simulink model "HQEV_MiL_20160830_integrate_r2017a_testframe"  (R2017a)
settings: Solver=FixedStepDiscrete  StartTime=0.0  StopTime=inf  FixedStep=0.01  RelTol=1e-3  EnableMultiTasking=on
PreLoadFcn:
  | try
  | load('HQEV_MiL_20160830_integrate_r2017a_testframe_tpt_so.mat');
  | catch
  | error('Could not load the file HQEV_MiL_20160830_integrate_r2017a_testframe_tpt_so.mat. This file contains Simulink objects that are possibly required for executing the test frame model. Try re-generating the test frame model.');
  | end
PostLoadFcn:
  | , if any(exist('dsrtsu_mdlpostloadfcn', 'file') == [2, 3, 6]), try dsrtsu_mdlpostloadfcn('Execute', bdroot); catch fprintf('Error in PostLoadFcn (dsrtsu_mdlpostloadfcn) for model "%s":\n %s\n', bdroot, lasterr); end, end,
values from neighbouring files (symbols this model uses):
  tpt_stepsize = builtin('double',0.01)    [HQEV_MiL_20160830_integrate_r20_tpt_io.m]
undefined symbols (not defined in the file or in its folder): pPUD_cnt_ACChItErrThd_C, pPUD_cnt_ACHeatItErrThd_C, pPUD_cnt_DCChItErrThd_C, pPUD_cnt_DCHeatItErrThd_C, pPUD_s_ACChrg1NoRespTiout_C, pPUD_s_ACChrg2NoRespTiout_C, pPUD_s_ACChrgPtcEnDly_C, pPUD_s_BMSOnNoRespTiout_C, pPUD_s_DCChrg1NoRespTiout_C, pPUD_s_DCChrg2NoRespTiout_C, pPUD_s_EgyCoorrChItRecoverDly_C, pPUD_s_EgyCoorrDlyRstCtr_C, pPUD_s_EgyCoorrNoRespTiout_C, pPUD_V_MotPwrVolt_C, pPUD_V_MotRpdDisVolt_C, PUD, PUD_lib
libraries: BaseOperationLib_Browser x22, simulink x1, tpt_sfun_lib x1
settings Model: Creator=wuaibin  LastModifiedBy=YangFuchun
settings DataIOCC: LimitDataPoints=on  SaveFormat=StructureWithTime  SignalLoggingSaveFormat=ModelDataLogs
settings OptimizationCC: BlockReduction=off  UseFloatMulNetSlope=on  DefaultUnderspecifiedDataType=single  ExpressionDepthLimit=2147483647  LifeSpan=inf
settings DebuggingCC: UnderspecifiedInitializationDetection=Classic  MergeDetectMultiDrivingBlocksExec=none  SolverPrmCheckMsg=warning  FcnCallInpInsideContextMsg=warning  StateNameClashWarn=warning  StrictBusMsg=ErrorOnBusTreatedAsVector  NonBusSignalsTreatedAsBus=error  SFUnexpectedBacktrackingDiag=warning  SFNoUnconditionalDefaultTransitionDiag=warning  SFExecutionAtInitializationDiag=none
settings HardwareCC: ProdBitPerPointer=32  ProdBitPerSizeT=32  ProdBitPerPtrDiffT=32  ProdLargestAtomicFloat=None  ProdEndianess=BigEndian  ProdWordSize=32  ProdHWDeviceType=Generic->Custom  TargetIntDivRoundTo=Zero  TargetEndianess=BigEndian  TargetHWDeviceType=Generic->Custom
settings ModelReferenceCC: PropagateSignalLabelsOutOfModel=off
settings RTWCC: GenerateMakefile=off  TemplateMakefile=grt_msvc.tmf  Description="Visual C/C++ Project Makefile only for the \"grt\" target"
settings GRTTargetCC: TargetLangStandard=C89/C90 (ANSI)  GeneratePreprocessorConditionals=Disable all  CombineOutputUpdateFcns=off  GRTInterface=on
settings ConfigComp: CovMetricSettings=dw  CovHtmlReporting=on  CovSaveCumulativeToWorkspaceVar=on  CovSaveSingleToWorkspaceVar=on  CovExternalEMLEnable=off  CovSFcnEnable=off

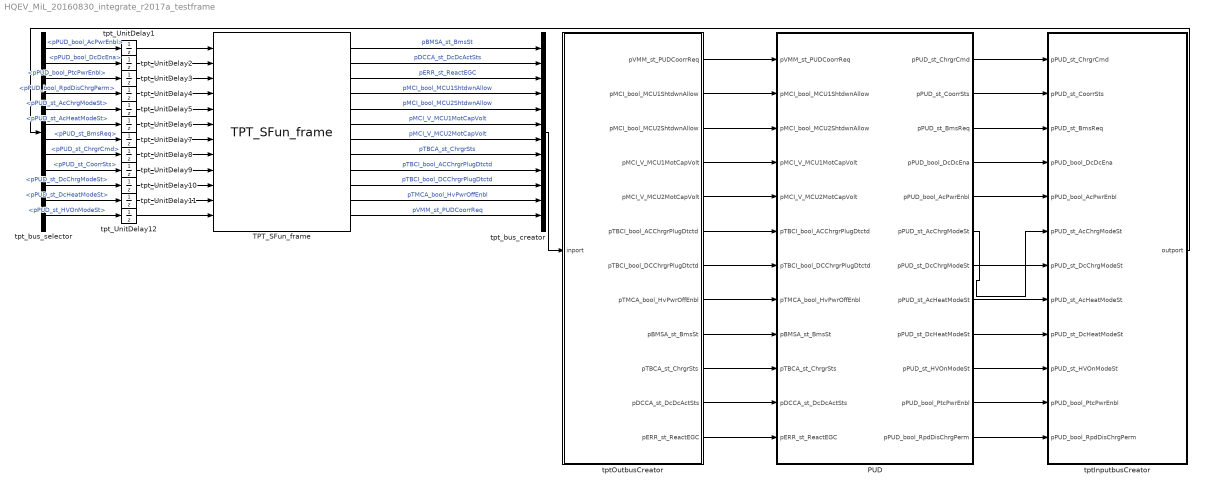
== system HQEV_MiL_20160830_integrate_r2017a_testframe ==
  PUD : Subsystem  AncestorBlock=PUD_lib/PUD  TreatAsAtomicUnit=on
  TPT_SFun_frame : tpt_sfun_lib/TPT_SFun_frame  tpt_inpDes=tpt_inpDes  tpt_outDes=tpt_outDes  tpt_progfile=tpt_progfile  tpt_binfile=tpt_binfile  tpt_stepsize=tpt_stepsize  tpt_stime_mode=Cyclic  tpt_localIOSig=char('pPUD_bool_AcPwrEnblboolean1pPUD_bool_DcDcEnaboolean1pPUD_bool_PtcPwrEnblboolean1pPUD_bool_RpdDisChrgPermboolean1pPUD_st_AcChrgModeStuint81pPUD_st_AcHeatModeStuint81pPUD_st_BmsRequint81pPUD_st_ChrgrCmduint81pPUD_st_CoorrStsuint81pPUD_st_DcChrgModeStuint81pPUD_st_DcHeatModeStuint81pPUD_st_HVOnModeStuint81pBMSA_st_BmsStuint81pDCCA_st_DcDcActStsuint81pERR_st_ReactEGCuint321pMCI_bool_MCU1ShtdwnAllowboolean1pMCI_bool_MCU2ShtdwnAllowboolean1pMCI_V_MCU1MotCapVoltfloat1pMCI_V_MCU2MotCapVoltfloat1pTBCA_st_ChrgrStsuint81pTBCI_bool_ACChrgrPlugDtctdboolean1pTBCI_bool_DCChrgrPlugDtctdboolean1pTMCA_bool_HvPwrOffEnblboolean1pVMM_st_PUDCoorrRequint81')  tpt_localSFunBuildTime=7.3699745777e+05
  tptInputbusCreator : Subsystem
  tptOutbusCreator : Subsystem
  tpt_UnitDelay{1..12} (12 alike) : UnitDelay  SampleTime=tpt_stepsize
  tpt_bus_creator : BusCreator  Inputs=12
  tpt_bus_selector : BusSelector  OutputSignals=pPUD_bool_AcPwrEnbl,pPUD_bool_DcDcEna,pPUD_bool_PtcPwrEnbl,pPUD_bool_RpdDisChrgPerm,pPUD_st_AcChrgModeSt,pPUD_st_AcHeatModeSt,pPUD_st_BmsReq,pPUD_st_ChrgrCmd,pPUD_st_CoorrSts,pPUD_st_DcChrgModeSt,pPUD_st_DcHeatModeSt,pPUD_st_HVOnModeSt
  wires:
  tpt_UnitDelay1/1 -> TPT_SFun_frame/1
  tpt_bus_selector/1 -> tpt_UnitDelay1/1  "<pPUD_bool_AcPwrEnbl>"
  tpt_UnitDelay2/1 -> TPT_SFun_frame/2
  tpt_bus_selector/2 -> tpt_UnitDelay2/1  "<pPUD_bool_DcDcEna>"
  tpt_UnitDelay3/1 -> TPT_SFun_frame/3
  tpt_bus_selector/3 -> tpt_UnitDelay3/1  "<pPUD_bool_PtcPwrEnbl>"
  tpt_UnitDelay4/1 -> TPT_SFun_frame/4
  tpt_bus_selector/4 -> tpt_UnitDelay4/1  "<pPUD_bool_RpdDisChrgPerm>"
  tpt_UnitDelay5/1 -> TPT_SFun_frame/5
  tpt_bus_selector/5 -> tpt_UnitDelay5/1  "<pPUD_st_AcChrgModeSt>"
  tpt_UnitDelay6/1 -> TPT_SFun_frame/6
  tpt_bus_selector/6 -> tpt_UnitDelay6/1  "<pPUD_st_AcHeatModeSt>"
  tpt_UnitDelay7/1 -> TPT_SFun_frame/7
  tpt_bus_selector/7 -> tpt_UnitDelay7/1  "<pPUD_st_BmsReq>"
  tpt_UnitDelay8/1 -> TPT_SFun_frame/8
  tpt_bus_selector/8 -> tpt_UnitDelay8/1  "<pPUD_st_ChrgrCmd>"
  tpt_UnitDelay9/1 -> TPT_SFun_frame/9
  tpt_bus_selector/9 -> tpt_UnitDelay9/1  "<pPUD_st_CoorrSts>"
  tpt_UnitDelay10/1 -> TPT_SFun_frame/10
  tpt_bus_selector/10 -> tpt_UnitDelay10/1  "<pPUD_st_DcChrgModeSt>"
  tpt_UnitDelay11/1 -> TPT_SFun_frame/11
  tpt_bus_selector/11 -> tpt_UnitDelay11/1  "<pPUD_st_DcHeatModeSt>"
  tpt_UnitDelay12/1 -> TPT_SFun_frame/12
  tpt_bus_selector/12 -> tpt_UnitDelay12/1  "<pPUD_st_HVOnModeSt>"
  TPT_SFun_frame/1 -> tpt_bus_creator/1  "pBMSA_st_BmsSt"
  TPT_SFun_frame/2 -> tpt_bus_creator/2  "pDCCA_st_DcDcActSts"
  TPT_SFun_frame/3 -> tpt_bus_creator/3  "pERR_st_ReactEGC"
  TPT_SFun_frame/4 -> tpt_bus_creator/4  "pMCI_bool_MCU1ShtdwnAllow"
  TPT_SFun_frame/5 -> tpt_bus_creator/5  "pMCI_bool_MCU2ShtdwnAllow"
  TPT_SFun_frame/6 -> tpt_bus_creator/6  "pMCI_V_MCU1MotCapVolt"
  TPT_SFun_frame/7 -> tpt_bus_creator/7  "pMCI_V_MCU2MotCapVolt"
  TPT_SFun_frame/8 -> tpt_bus_creator/8  "pTBCA_st_ChrgrSts"
  TPT_SFun_frame/9 -> tpt_bus_creator/9  "pTBCI_bool_ACChrgrPlugDtctd"
  TPT_SFun_frame/10 -> tpt_bus_creator/10  "pTBCI_bool_DCChrgrPlugDtctd"
  TPT_SFun_frame/11 -> tpt_bus_creator/11  "pTMCA_bool_HvPwrOffEnbl"
  TPT_SFun_frame/12 -> tpt_bus_creator/12  "pVMM_st_PUDCoorrReq"
  tpt_bus_creator/1 -> tptOutbusCreator/1(inport)
  tptOutbusCreator/1(pVMM_st_PUDCoorrReq) -> PUD/1(pVMM_st_PUDCoorrReq)
  tptOutbusCreator/2(pMCI_bool_MCU1ShtdwnAllow) -> PUD/2(pMCI_bool_MCU1ShtdwnAllow)
  tptOutbusCreator/3(pMCI_bool_MCU2ShtdwnAllow) -> PUD/3(pMCI_bool_MCU2ShtdwnAllow)
  tptOutbusCreator/4(pMCI_V_MCU1MotCapVolt) -> PUD/4(pMCI_V_MCU1MotCapVolt)
  tptOutbusCreator/5(pMCI_V_MCU2MotCapVolt) -> PUD/5(pMCI_V_MCU2MotCapVolt)
  tptOutbusCreator/6(pTBCI_bool_ACChrgrPlugDtctd) -> PUD/6(pTBCI_bool_ACChrgrPlugDtctd)
  tptOutbusCreator/7(pTBCI_bool_DCChrgrPlugDtctd) -> PUD/7(pTBCI_bool_DCChrgrPlugDtctd)
  tptOutbusCreator/8(pTMCA_bool_HvPwrOffEnbl) -> PUD/8(pTMCA_bool_HvPwrOffEnbl)
  tptOutbusCreator/9(pBMSA_st_BmsSt) -> PUD/9(pBMSA_st_BmsSt)
  tptOutbusCreator/10(pTBCA_st_ChrgrSts) -> PUD/10(pTBCA_st_ChrgrSts)
  tptOutbusCreator/11(pDCCA_st_DcDcActSts) -> PUD/11(pDCCA_st_DcDcActSts)
  tptOutbusCreator/12(pERR_st_ReactEGC) -> PUD/12(pERR_st_ReactEGC)
  PUD/1(pPUD_st_ChrgrCmd) -> tptInputbusCreator/1(pPUD_st_ChrgrCmd)
  PUD/2(pPUD_st_CoorrSts) -> tptInputbusCreator/2(pPUD_st_CoorrSts)
  PUD/3(pPUD_st_BmsReq) -> tptInputbusCreator/3(pPUD_st_BmsReq)
  PUD/4(pPUD_bool_DcDcEna) -> tptInputbusCreator/4(pPUD_bool_DcDcEna)
  PUD/5(pPUD_bool_AcPwrEnbl) -> tptInputbusCreator/5(pPUD_bool_AcPwrEnbl)
  PUD/6(pPUD_st_AcChrgModeSt) -> tptInputbusCreator/6(pPUD_st_AcChrgModeSt)
  PUD/7(pPUD_st_DcChrgModeSt) -> tptInputbusCreator/7(pPUD_st_DcChrgModeSt)
  PUD/8(pPUD_st_AcHeatModeSt) -> tptInputbusCreator/8(pPUD_st_AcHeatModeSt)
  PUD/9(pPUD_st_DcHeatModeSt) -> tptInputbusCreator/9(pPUD_st_DcHeatModeSt)
  PUD/10(pPUD_st_HVOnModeSt) -> tptInputbusCreator/10(pPUD_st_HVOnModeSt)
  PUD/11(pPUD_bool_PtcPwrEnbl) -> tptInputbusCreator/11(pPUD_bool_PtcPwrEnbl)
  PUD/12(pPUD_bool_RpdDisChrgPerm) -> tptInputbusCreator/12(pPUD_bool_RpdDisChrgPerm)
  tptInputbusCreator/1(outport) -> tpt_bus_selector/1

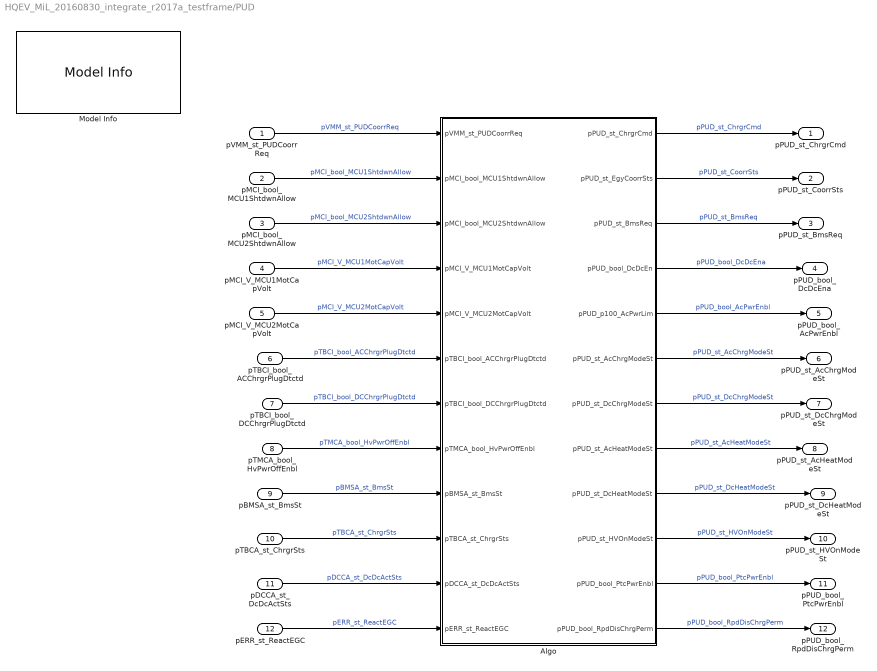
== system HQEV_MiL_20160830_integrate_r2017a_testframe/PUD ==
  pVMM_st_PUDCoorrReq : Inport
  pMCI_bool_MCU1ShtdwnAllow : Inport  Port=2
  pMCI_bool_MCU2ShtdwnAllow : Inport  Port=3
  pMCI_V_MCU1MotCapVolt : Inport  Port=4
  pMCI_V_MCU2MotCapVolt : Inport  Port=5
  pTBCI_bool_ACChrgrPlugDtctd : Inport  Port=6
  pTBCI_bool_DCChrgrPlugDtctd : Inport  Port=7
  pTMCA_bool_HvPwrOffEnbl : Inport  Port=8  OutDataTypeStr=boolean
  pBMSA_st_BmsSt : Inport  Port=9
  pTBCA_st_ChrgrSts : Inport  Port=10
  pDCCA_st_DcDcActSts : Inport  Port=11
  pERR_st_ReactEGC : Inport  Port=12
  Algo : Subsystem
  Model Info : simulink/Model-Wide Utilities/Model Info  InitialBlockCM=None  BlockCM=None  Frame=on  DisplayStringWithTags=Model Info\nCreated: %<Created>\nCreator: wuaibin  HorizontalTextAlignment=Center  LeftAlignmentValue=0.5  SourceBlockDiagram=HQEV_HCU  TagMaxNumber=20
  pPUD_st_ChrgrCmd : Outport
  pPUD_st_CoorrSts : Outport  Port=2
  pPUD_st_BmsReq : Outport  Port=3
  pPUD_bool_DcDcEna : Outport  Port=4
  pPUD_bool_AcPwrEnbl : Outport  Port=5
  pPUD_st_AcChrgModeSt : Outport  Port=6
  pPUD_st_DcChrgModeSt : Outport  Port=7
  pPUD_st_AcHeatModeSt : Outport  Port=8
  pPUD_st_DcHeatModeSt : Outport  Port=9
  pPUD_st_HVOnModeSt : Outport  Port=10
  pPUD_bool_PtcPwrEnbl : Outport  Port=11
  pPUD_bool_RpdDisChrgPerm : Outport  Port=12
  wires:
  pTBCI_bool_DCChrgrPlugDtctd/1 -> Algo/7(pTBCI_bool_DCChrgrPlugDtctd)  "pTBCI_bool_DCChrgrPlugDtctd"
  pTBCI_bool_ACChrgrPlugDtctd/1 -> Algo/6(pTBCI_bool_ACChrgrPlugDtctd)  "pTBCI_bool_ACChrgrPlugDtctd"
  pVMM_st_PUDCoorrReq/1 -> Algo/1(pVMM_st_PUDCoorrReq)  "pVMM_st_PUDCoorrReq"
  pMCI_bool_MCU1ShtdwnAllow/1 -> Algo/2(pMCI_bool_MCU1ShtdwnAllow)  "pMCI_bool_MCU1ShtdwnAllow"
  pMCI_bool_MCU2ShtdwnAllow/1 -> Algo/3(pMCI_bool_MCU2ShtdwnAllow)  "pMCI_bool_MCU2ShtdwnAllow"
  pTMCA_bool_HvPwrOffEnbl/1 -> Algo/8(pTMCA_bool_HvPwrOffEnbl)  "pTMCA_bool_HvPwrOffEnbl"
  pBMSA_st_BmsSt/1 -> Algo/9(pBMSA_st_BmsSt)  "pBMSA_st_BmsSt"
  pTBCA_st_ChrgrSts/1 -> Algo/10(pTBCA_st_ChrgrSts)  "pTBCA_st_ChrgrSts"
  pDCCA_st_DcDcActSts/1 -> Algo/11(pDCCA_st_DcDcActSts)  "pDCCA_st_DcDcActSts"
  Algo/1(pPUD_st_ChrgrCmd) -> pPUD_st_ChrgrCmd/1  "pPUD_st_ChrgrCmd"
  Algo/2(pPUD_st_EgyCoorrSts) -> pPUD_st_CoorrSts/1  "pPUD_st_CoorrSts"
  Algo/3(pPUD_st_BmsReq) -> pPUD_st_BmsReq/1  "pPUD_st_BmsReq"
  Algo/4(pPUD_bool_DcDcEn) -> pPUD_bool_DcDcEna/1  "pPUD_bool_DcDcEna"
  Algo/5(pPUD_p100_AcPwrLim) -> pPUD_bool_AcPwrEnbl/1  "pPUD_bool_AcPwrEnbl"
  Algo/6(pPUD_st_AcChrgModeSt) -> pPUD_st_AcChrgModeSt/1  "pPUD_st_AcChrgModeSt"
  Algo/7(pPUD_st_DcChrgModeSt) -> pPUD_st_DcChrgModeSt/1  "pPUD_st_DcChrgModeSt"
  Algo/8(pPUD_st_AcHeatModeSt) -> pPUD_st_AcHeatModeSt/1  "pPUD_st_AcHeatModeSt"
  Algo/9(pPUD_st_DcHeatModeSt) -> pPUD_st_DcHeatModeSt/1  "pPUD_st_DcHeatModeSt"
  Algo/10(pPUD_st_HVOnModeSt) -> pPUD_st_HVOnModeSt/1  "pPUD_st_HVOnModeSt"
  Algo/11(pPUD_bool_PtcPwrEnbl) -> pPUD_bool_PtcPwrEnbl/1  "pPUD_bool_PtcPwrEnbl"
  pMCI_V_MCU1MotCapVolt/1 -> Algo/4(pMCI_V_MCU1MotCapVolt)  "pMCI_V_MCU1MotCapVolt"
  pMCI_V_MCU2MotCapVolt/1 -> Algo/5(pMCI_V_MCU2MotCapVolt)  "pMCI_V_MCU2MotCapVolt"
  Algo/12(pPUD_bool_RpdDisChrgPerm) -> pPUD_bool_RpdDisChrgPerm/1  "pPUD_bool_RpdDisChrgPerm"
  pERR_st_ReactEGC/1 -> Algo/12(pERR_st_ReactEGC)  "pERR_st_ReactEGC"

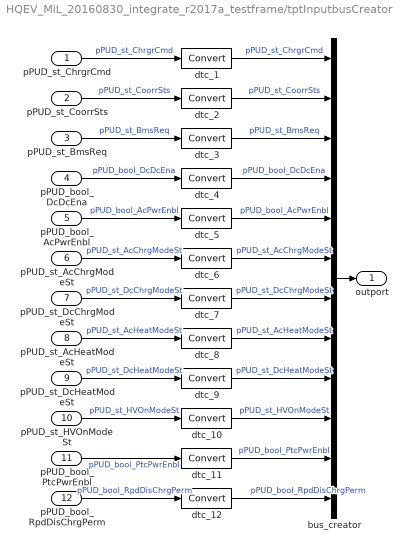
== system HQEV_MiL_20160830_integrate_r2017a_testframe/tptInputbusCreator ==
  pPUD_st_ChrgrCmd : Inport
  pPUD_st_CoorrSts : Inport  Port=2
  pPUD_st_BmsReq : Inport  Port=3
  pPUD_bool_DcDcEna : Inport  Port=4
  pPUD_bool_AcPwrEnbl : Inport  Port=5
  pPUD_st_AcChrgModeSt : Inport  Port=6
  pPUD_st_DcChrgModeSt : Inport  Port=7
  pPUD_st_AcHeatModeSt : Inport  Port=8
  pPUD_st_DcHeatModeSt : Inport  Port=9
  pPUD_st_HVOnModeSt : Inport  Port=10
  pPUD_bool_PtcPwrEnbl : Inport  Port=11
  pPUD_bool_RpdDisChrgPerm : Inport  Port=12
  bus_creator : BusCreator  Inputs=12
  dtc_{1..12} (12 alike) : DataTypeConversion  SaturateOnIntegerOverflow=on  RndMeth=Zero
  outport : Outport
  wires:
  bus_creator/1 -> outport/1
  dtc_1/1 -> bus_creator/1  "pPUD_st_ChrgrCmd"
  dtc_2/1 -> bus_creator/2  "pPUD_st_CoorrSts"
  dtc_3/1 -> bus_creator/3  "pPUD_st_BmsReq"
  dtc_4/1 -> bus_creator/4  "pPUD_bool_DcDcEna"
  dtc_5/1 -> bus_creator/5  "pPUD_bool_AcPwrEnbl"
  dtc_6/1 -> bus_creator/6  "pPUD_st_AcChrgModeSt"
  dtc_7/1 -> bus_creator/7  "pPUD_st_DcChrgModeSt"
  dtc_8/1 -> bus_creator/8  "pPUD_st_AcHeatModeSt"
  dtc_9/1 -> bus_creator/9  "pPUD_st_DcHeatModeSt"
  dtc_10/1 -> bus_creator/10  "pPUD_st_HVOnModeSt"
  dtc_11/1 -> bus_creator/11  "pPUD_bool_PtcPwrEnbl"
  dtc_12/1 -> bus_creator/12  "pPUD_bool_RpdDisChrgPerm"
  pPUD_st_ChrgrCmd/1 -> dtc_1/1  "pPUD_st_ChrgrCmd"
  pPUD_st_CoorrSts/1 -> dtc_2/1  "pPUD_st_CoorrSts"
  pPUD_st_BmsReq/1 -> dtc_3/1  "pPUD_st_BmsReq"
  pPUD_bool_DcDcEna/1 -> dtc_4/1  "pPUD_bool_DcDcEna"
  pPUD_bool_AcPwrEnbl/1 -> dtc_5/1  "pPUD_bool_AcPwrEnbl"
  pPUD_st_AcChrgModeSt/1 -> dtc_6/1  "pPUD_st_AcChrgModeSt"
  pPUD_st_DcChrgModeSt/1 -> dtc_7/1  "pPUD_st_DcChrgModeSt"
  pPUD_st_AcHeatModeSt/1 -> dtc_8/1  "pPUD_st_AcHeatModeSt"
  pPUD_st_DcHeatModeSt/1 -> dtc_9/1  "pPUD_st_DcHeatModeSt"
  pPUD_st_HVOnModeSt/1 -> dtc_10/1  "pPUD_st_HVOnModeSt"
  pPUD_bool_PtcPwrEnbl/1 -> dtc_11/1  "pPUD_bool_PtcPwrEnbl"
  pPUD_bool_RpdDisChrgPerm/1 -> dtc_12/1  "pPUD_bool_RpdDisChrgPerm"

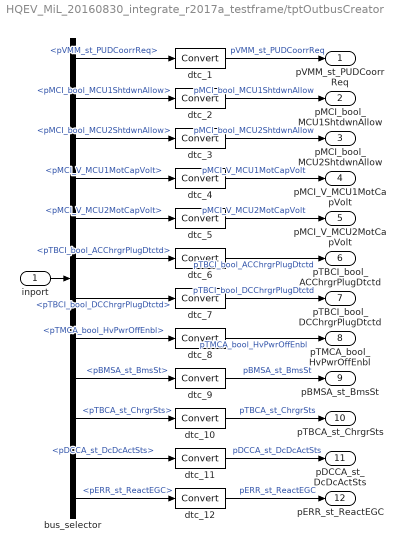
== system HQEV_MiL_20160830_integrate_r2017a_testframe/tptOutbusCreator ==
  inport : Inport
  bus_selector : BusSelector  OutputSignals=pVMM_st_PUDCoorrReq,pMCI_bool_MCU1ShtdwnAllow,pMCI_bool_MCU2ShtdwnAllow,pMCI_V_MCU1MotCapVolt,pMCI_V_MCU2MotCapVolt,pTBCI_bool_ACChrgrPlugDtctd,pTBCI_bool_DCChrgrPlugDtctd,pTMCA_bool_HvPwrOffEnbl,pBMSA_st_BmsSt,pTBCA_st_ChrgrSts,pDCCA_st_DcDcActSts,pERR_st_ReactEGC
  dtc_{1..12} (12 alike) : DataTypeConversion  SaturateOnIntegerOverflow=on  RndMeth=Zero
  pVMM_st_PUDCoorrReq : Outport
  pMCI_bool_MCU1ShtdwnAllow : Outport  Port=2
  pMCI_bool_MCU2ShtdwnAllow : Outport  Port=3
  pMCI_V_MCU1MotCapVolt : Outport  Port=4
  pMCI_V_MCU2MotCapVolt : Outport  Port=5
  pTBCI_bool_ACChrgrPlugDtctd : Outport  Port=6
  pTBCI_bool_DCChrgrPlugDtctd : Outport  Port=7
  pTMCA_bool_HvPwrOffEnbl : Outport  Port=8
  pBMSA_st_BmsSt : Outport  Port=9
  pTBCA_st_ChrgrSts : Outport  Port=10
  pDCCA_st_DcDcActSts : Outport  Port=11
  pERR_st_ReactEGC : Outport  Port=12
  wires:
  inport/1 -> bus_selector/1
  bus_selector/1 -> dtc_1/1  "<pVMM_st_PUDCoorrReq>"
  bus_selector/2 -> dtc_2/1  "<pMCI_bool_MCU1ShtdwnAllow>"
  bus_selector/3 -> dtc_3/1  "<pMCI_bool_MCU2ShtdwnAllow>"
  bus_selector/4 -> dtc_4/1  "<pMCI_V_MCU1MotCapVolt>"
  bus_selector/5 -> dtc_5/1  "<pMCI_V_MCU2MotCapVolt>"
  bus_selector/6 -> dtc_6/1  "<pTBCI_bool_ACChrgrPlugDtctd>"
  bus_selector/7 -> dtc_7/1  "<pTBCI_bool_DCChrgrPlugDtctd>"
  bus_selector/8 -> dtc_8/1  "<pTMCA_bool_HvPwrOffEnbl>"
  bus_selector/9 -> dtc_9/1  "<pBMSA_st_BmsSt>"
  bus_selector/10 -> dtc_10/1  "<pTBCA_st_ChrgrSts>"
  bus_selector/11 -> dtc_11/1  "<pDCCA_st_DcDcActSts>"
  bus_selector/12 -> dtc_12/1  "<pERR_st_ReactEGC>"
  dtc_1/1 -> pVMM_st_PUDCoorrReq/1  "pVMM_st_PUDCoorrReq"
  dtc_2/1 -> pMCI_bool_MCU1ShtdwnAllow/1  "pMCI_bool_MCU1ShtdwnAllow"
  dtc_3/1 -> pMCI_bool_MCU2ShtdwnAllow/1  "pMCI_bool_MCU2ShtdwnAllow"
  dtc_4/1 -> pMCI_V_MCU1MotCapVolt/1  "pMCI_V_MCU1MotCapVolt"
  dtc_5/1 -> pMCI_V_MCU2MotCapVolt/1  "pMCI_V_MCU2MotCapVolt"
  dtc_6/1 -> pTBCI_bool_ACChrgrPlugDtctd/1  "pTBCI_bool_ACChrgrPlugDtctd"
  dtc_7/1 -> pTBCI_bool_DCChrgrPlugDtctd/1  "pTBCI_bool_DCChrgrPlugDtctd"
  dtc_8/1 -> pTMCA_bool_HvPwrOffEnbl/1  "pTMCA_bool_HvPwrOffEnbl"
  dtc_9/1 -> pBMSA_st_BmsSt/1  "pBMSA_st_BmsSt"
  dtc_10/1 -> pTBCA_st_ChrgrSts/1  "pTBCA_st_ChrgrSts"
  dtc_11/1 -> pDCCA_st_DcDcActSts/1  "pDCCA_st_DcDcActSts"
  dtc_12/1 -> pERR_st_ReactEGC/1  "pERR_st_ReactEGC"

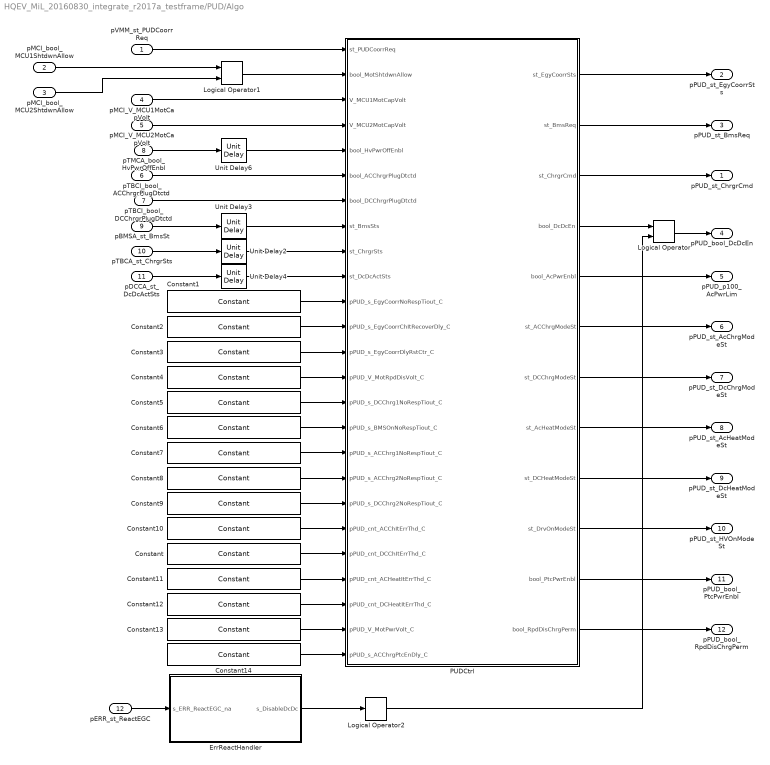
== system HQEV_MiL_20160830_integrate_r2017a_testframe/PUD/Algo ==
  pVMM_st_PUDCoorrReq : Inport
  pMCI_bool_MCU1ShtdwnAllow : Inport  Port=2
  pMCI_bool_MCU2ShtdwnAllow : Inport  Port=3
  pMCI_V_MCU1MotCapVolt : Inport  Port=4
  pMCI_V_MCU2MotCapVolt : Inport  Port=5
  pTBCI_bool_ACChrgrPlugDtctd : Inport  Port=6
  pTBCI_bool_DCChrgrPlugDtctd : Inport  Port=7
  pTMCA_bool_HvPwrOffEnbl : Inport  Port=8
  pBMSA_st_BmsSt : Inport  Port=9
  pTBCA_st_ChrgrSts : Inport  Port=10
  pDCCA_st_DcDcActSts : Inport  Port=11
  pERR_st_ReactEGC : Inport  Port=12
  Constant : BaseOperationLib_Browser/Sources&Sinks/Constant  Value=pPUD_cnt_DCChItErrThd_C  OutMin=[]  OutMax=[]  OutDataTypeStr=Inherit: Inherit from 'Constant value'
  Constant1 : BaseOperationLib_Browser/Sources&Sinks/Constant  Value=pPUD_s_EgyCoorrNoRespTiout_C  OutMin=[]  OutMax=[]  OutDataTypeStr=Inherit: Inherit from 'Constant value'
  Constant10 : BaseOperationLib_Browser/Sources&Sinks/Constant  Value=pPUD_cnt_ACChItErrThd_C  OutMin=[]  OutMax=[]  OutDataTypeStr=Inherit: Inherit from 'Constant value'
  Constant11 : BaseOperationLib_Browser/Sources&Sinks/Constant  Value=pPUD_cnt_ACHeatItErrThd_C  OutMin=[]  OutMax=[]  OutDataTypeStr=Inherit: Inherit from 'Constant value'
  Constant12 : BaseOperationLib_Browser/Sources&Sinks/Constant  Value=pPUD_cnt_DCHeatItErrThd_C  OutMin=[]  OutMax=[]  OutDataTypeStr=Inherit: Inherit from 'Constant value'
  Constant13 : BaseOperationLib_Browser/Sources&Sinks/Constant  Value=pPUD_V_MotPwrVolt_C  OutMin=[]  OutMax=[]  OutDataTypeStr=Inherit: Inherit from 'Constant value'
  Constant14 : BaseOperationLib_Browser/Sources&Sinks/Constant  Value=pPUD_s_ACChrgPtcEnDly_C  OutMin=[]  OutMax=[]  OutDataTypeStr=Inherit: Inherit from 'Constant value'
  Constant2 : BaseOperationLib_Browser/Sources&Sinks/Constant  Value=pPUD_s_EgyCoorrChItRecoverDly_C  OutMin=[]  OutMax=[]  OutDataTypeStr=Inherit: Inherit from 'Constant value'
  Constant3 : BaseOperationLib_Browser/Sources&Sinks/Constant  Value=pPUD_s_EgyCoorrDlyRstCtr_C  OutMin=[]  OutMax=[]  OutDataTypeStr=Inherit: Inherit from 'Constant value'
  Constant4 : BaseOperationLib_Browser/Sources&Sinks/Constant  Value=pPUD_V_MotRpdDisVolt_C  OutMin=[]  OutMax=[]  OutDataTypeStr=Inherit: Inherit from 'Constant value'
  Constant5 : BaseOperationLib_Browser/Sources&Sinks/Constant  Value=pPUD_s_DCChrg1NoRespTiout_C  OutMin=[]  OutMax=[]  OutDataTypeStr=Inherit: Inherit from 'Constant value'
  Constant6 : BaseOperationLib_Browser/Sources&Sinks/Constant  Value=pPUD_s_BMSOnNoRespTiout_C  VectorParams1D=off  OutMin=[]  OutMax=[]  OutDataTypeStr=Inherit: Inherit from 'Constant value'
  Constant7 : BaseOperationLib_Browser/Sources&Sinks/Constant  Value=pPUD_s_ACChrg1NoRespTiout_C  OutMin=[]  OutMax=[]  OutDataTypeStr=Inherit: Inherit from 'Constant value'
  Constant8 : BaseOperationLib_Browser/Sources&Sinks/Constant  Value=pPUD_s_ACChrg2NoRespTiout_C  OutMin=[]  OutMax=[]  OutDataTypeStr=Inherit: Inherit from 'Constant value'
  Constant9 : BaseOperationLib_Browser/Sources&Sinks/Constant  Value=pPUD_s_DCChrg2NoRespTiout_C  OutMin=[]  OutMax=[]  OutDataTypeStr=Inherit: Inherit from 'Constant value'
  ErrReactHandler : Subsystem
  Logical Operator : BaseOperationLib_Browser/Logic Operations Changed/Logical Operator  Operator=AND  Inputs=2  AllPortsSameDT=off  OutDataTypeStr=boolean
  Logical Operator1 : BaseOperationLib_Browser/Logic Operations Changed/Logical Operator  Operator=AND  Inputs=2  AllPortsSameDT=off  OutDataTypeStr=boolean
  Logical Operator2 : BaseOperationLib_Browser/Logic Operations Changed/Logical Operator  Operator=NOT  Inputs=2  AllPortsSameDT=off  OutDataTypeStr=boolean
  PUDCtrl : Stateflow chart  TreatAsAtomicUnit=on
  Unit Delay{2..4,6} (4 alike) : BaseOperationLib_Browser/Discrete Unchanged /Unit Delay  InitialCondition=0  InputProcessing=Inherited  SampleTime=-1
  pPUD_st_ChrgrCmd : Outport
  pPUD_st_EgyCoorrSts : Outport  Port=2
  pPUD_st_BmsReq : Outport  Port=3
  pPUD_bool_DcDcEn : Outport  Port=4
  pPUD_p100_AcPwrLim : Outport  Port=5
  pPUD_st_AcChrgModeSt : Outport  Port=6
  pPUD_st_DcChrgModeSt : Outport  Port=7
  pPUD_st_AcHeatModeSt : Outport  Port=8
  pPUD_st_DcHeatModeSt : Outport  Port=9
  pPUD_st_HVOnModeSt : Outport  Port=10
  pPUD_bool_PtcPwrEnbl : Outport  Port=11
  pPUD_bool_RpdDisChrgPerm : Outport  Port=12
  wires:
  Constant14/1 -> PUDCtrl/25(pPUD_s_ACChrgPtcEnDly_C)
  Constant13/1 -> PUDCtrl/24(pPUD_V_MotPwrVolt_C)
  pTBCI_bool_DCChrgrPlugDtctd/1 -> PUDCtrl/7(bool_DCChrgrPlugDtctd)
  pTBCI_bool_ACChrgrPlugDtctd/1 -> PUDCtrl/6(bool_ACChrgrPlugDtctd)
  PUDCtrl/4(bool_DcDcEn) -> Logical Operator/1
  pDCCA_st_DcDcActSts/1 -> Unit Delay4/1
  pVMM_st_PUDCoorrReq/1 -> PUDCtrl/1(st_PUDCoorrReq)
  PUDCtrl/1(st_EgyCoorrSts) -> pPUD_st_EgyCoorrSts/1
  PUDCtrl/2(st_BmsReq) -> pPUD_st_BmsReq/1
  PUDCtrl/3(st_ChrgrCmd) -> pPUD_st_ChrgrCmd/1
  pBMSA_st_BmsSt/1 -> Unit Delay3/1
  pTBCA_st_ChrgrSts/1 -> Unit Delay2/1
  PUDCtrl/5(bool_AcPwrEnbl) -> pPUD_p100_AcPwrLim/1
  pTMCA_bool_HvPwrOffEnbl/1 -> Unit Delay6/1
  PUDCtrl/6(st_ACChrgModeSt) -> pPUD_st_AcChrgModeSt/1
  PUDCtrl/7(st_DCChrgModeSt) -> pPUD_st_DcChrgModeSt/1
  PUDCtrl/8(st_AcHeatModeSt) -> pPUD_st_AcHeatModeSt/1
  PUDCtrl/9(st_DCHeatModeSt) -> pPUD_st_DcHeatModeSt/1
  PUDCtrl/10(st_DrvOnModeSt) -> pPUD_st_HVOnModeSt/1
  PUDCtrl/11(bool_PtcPwrEnbl) -> pPUD_bool_PtcPwrEnbl/1
  Unit Delay6/1 -> PUDCtrl/5(bool_HvPwrOffEnbl)
  Unit Delay3/1 -> PUDCtrl/8(st_BmsSts)
  Unit Delay2/1 -> PUDCtrl/9(st_ChrgrSts)
  Unit Delay4/1 -> PUDCtrl/10(st_DcDcActSts)
  pMCI_bool_MCU2ShtdwnAllow/1 -> Logical Operator1/2
  pMCI_bool_MCU1ShtdwnAllow/1 -> Logical Operator1/1
  Logical Operator1/1 -> PUDCtrl/2(bool_MotShtdwnAllow)
  pMCI_V_MCU1MotCapVolt/1 -> PUDCtrl/3(V_MCU1MotCapVolt)
  pMCI_V_MCU2MotCapVolt/1 -> PUDCtrl/4(V_MCU2MotCapVolt)
  PUDCtrl/12(bool_RpdDisChrgPerm) -> pPUD_bool_RpdDisChrgPerm/1
  Logical Operator/1 -> pPUD_bool_DcDcEn/1
  ErrReactHandler/1(s_DisableDcDc) -> Logical Operator2/1
  pERR_st_ReactEGC/1 -> ErrReactHandler/1(s_ERR_ReactEGC_na)
  Constant/1 -> PUDCtrl/21(pPUD_cnt_DCChItErrThd_C)
  Constant1/1 -> PUDCtrl/11(pPUD_s_EgyCoorrNoRespTiout_C)
  Constant2/1 -> PUDCtrl/12(pPUD_s_EgyCoorrChItRecoverDly_C)
  Constant3/1 -> PUDCtrl/13(pPUD_s_EgyCoorrDlyRstCtr_C)
  Constant4/1 -> PUDCtrl/14(pPUD_V_MotRpdDisVolt_C)
  Constant5/1 -> PUDCtrl/15(pPUD_s_DCChrg1NoRespTiout_C)
  Constant6/1 -> PUDCtrl/16(pPUD_s_BMSOnNoRespTiout_C)
  Constant7/1 -> PUDCtrl/17(pPUD_s_ACChrg1NoRespTiout_C)
  Constant8/1 -> PUDCtrl/18(pPUD_s_ACChrg2NoRespTiout_C)
  Constant9/1 -> PUDCtrl/19(pPUD_s_DCChrg2NoRespTiout_C)
  Constant10/1 -> PUDCtrl/20(pPUD_cnt_ACChItErrThd_C)
  Constant11/1 -> PUDCtrl/22(pPUD_cnt_ACHeatItErrThd_C)
  Constant12/1 -> PUDCtrl/23(pPUD_cnt_DCHeatItErrThd_C)
  Logical Operator2/1 -> Logical Operator/2

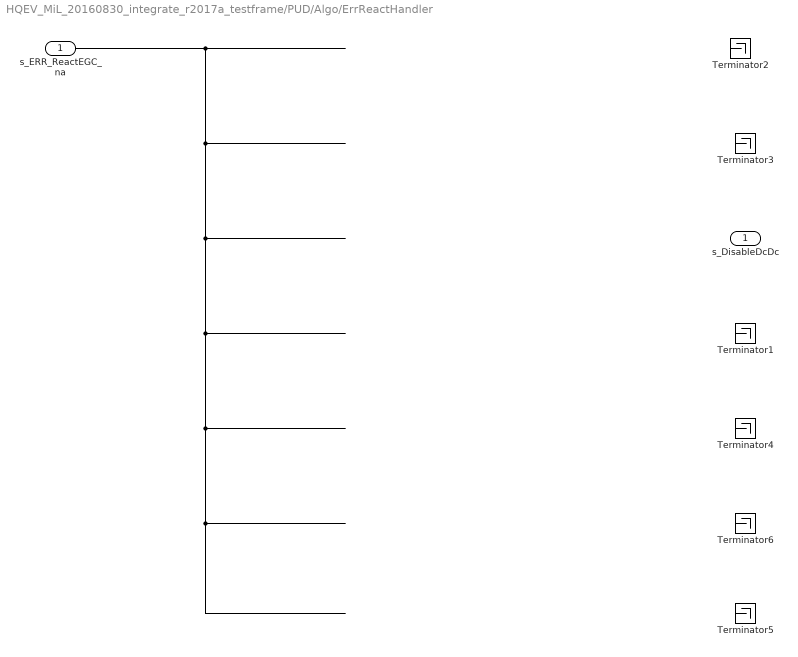
== system HQEV_MiL_20160830_integrate_r2017a_testframe/PUD/Algo/ErrReactHandler ==
  s_ERR_ReactEGC_na : Inport
  Terminator{1..6} (6 alike) : Terminator
  s_DisableDcDc : Outport
  wires:
  ? -> s_DisableDcDc/1
  ? -> Terminator2/1
  ? -> Terminator1/1
  ? -> Terminator4/1
  ? -> Terminator5/1
  s_ERR_ReactEGC_na/1 -> ?
  ? -> Terminator3/1
  ? -> Terminator6/1

== stateflow chart HQEV_MiL_20160830_integrate_r2017a_testframe/PUD/Algo/PUDCtrl ==
  state Normal
    state HVOff
      entry:
      st_EgyCoorrSts = PUDCoorrStsTyp.PUD_HVOFF;
      settings: description=HV off state. BMS is in HVoff or Shutdown state, depending on the operation mode (clamp status). If ignition is off the BMS is commanded to shutdown, if ignition is on it only goes to HVoff. This decision is made in the SetBMSCmd function.
      state HV_OFF [parallel]
        settings: executionOrder=1
        state ChargerInit
          entry:
          st_ChrgrCmd = ChrgrCmdTyp.STOP;
          ChItCtr = 0;
          SlaveNoResponse = 0;
        state HVAccStop
          entry:
          bool_DcDcEn = false;
          bool_AcPwrEnbl = false;
          bool_PtcPwrEnbl = false;
        state Motor_ShtDwn
        state BmsOff
          entry:
          st_BmsReq = uint8(BMSCmdTyp.BMS_CMD_HVOFF);
        state RapidDischarge
          entry:
          bool_RpdDisChrgPerm = true;
          exit:
          bool_RpdDisChrgPerm = false;
        state HvOff_ERR
          entry:
          st_EgyCoorrSts = PUDCoorrStsTyp.PUD_HVOFF_ERR;
        state HvOff
          entry:
          st_EgyCoorrSts = PUDCoorrStsTyp.PUD_HVOFF_OK;
        (default) -> Normal.HVOff.HV_OFF.ChargerInit
        Normal.HVOff.HV_OFF.ChargerInit -> HVAccStop : [st_ChrgrSts == ChrgrStsTyp.CST_STOP]
        HVAccStop -> Normal.HVOff.HV_OFF.Motor_ShtDwn : [st_DcDcActSts ==DCDCAStsTyp.DST_ShutDown && ...
            | bool_HvPwrOffEnbl == true || ...
            | after(pPUD_s_EgyCoorrNoRespTiout_C,sec)]
        Normal.HVOff.HV_OFF.Motor_ShtDwn -> BmsOff : [bool_MotShtdwnAllow == true]
        BmsOff -> Normal.HVOff.HV_OFF.HvOff_ERR [order 2] : [st_BmsSts == BMSStsTyp.BMS_HVOFF_ERR]
        BmsOff -> Normal.HVOff.HV_OFF.RapidDischarge [order 1] : [st_BmsSts == BMSStsTyp.BMS_HVOFF_OK]
        Normal.HVOff.HV_OFF.HvOff_ERR -> Normal.HVOff.HV_OFF.HvOff : [V_MCU1MotCapVolt < pPUD_V_MotRpdDisVolt_C && ...
            | V_MCU2MotCapVolt < pPUD_V_MotRpdDisVolt_C ]
        Normal.HVOff.HV_OFF.RapidDischarge -> Normal.HVOff.HV_OFF.HvOff : [V_MCU1MotCapVolt < pPUD_V_MotRpdDisVolt_C && ...
            | V_MCU2MotCapVolt < pPUD_V_MotRpdDisVolt_C ]
      state Chrg_Check [parallel]
        settings: executionOrder=2
        (default) -> (junction 3574)
        (junction 3574) -> (junction 3577) [order 1] : [bool_ACChrgrPlugDtctd == false && ...
            | bool_DCChrgrPlugDtctd == false]
        (junction 3574) -> (junction 3576) [order 2]
        (junction 3577) -> (junction 3578) : {
            | st_AcHeatModeSt = ACHeatModeTyp.PUD_ACHeat_Init;
            | st_ACChrgModeSt = ACChrgModeTyp.PUD_ACChrg_Init;
            | st_DCChrgModeSt = DCHeatModeTyp.PUD_DCHeat_Init;
            | st_DCChrgModeSt = DCChrgModeTyp.PUD_DCChrg_Init;
            | }
        (junction 3576) -> (junction 3579) [order 1] : [bool_ACChrgrPlugDtctd == false]
        (junction 3576) -> (junction 3593) [order 2]
        (junction 3579) -> (junction 3580) : {
            | st_AcHeatModeSt = ACHeatModeTyp.PUD_ACHeat_Init;
            | st_ACChrgModeSt = ACChrgModeTyp.PUD_ACChrg_Init;
            | }
        (junction 3593) -> (junction 3592) [order 1] : [bool_DCChrgrPlugDtctd == false]
        (junction 3593) -> (junction 3575) [order 2]
        (junction 3592) -> (junction 3596) : {
            | st_DCChrgModeSt = DCHeatModeTyp.PUD_DCHeat_Init;
            | st_DCChrgModeSt = DCChrgModeTyp.PUD_DCChrg_Init;
            | }
        (junction 3596) -> (junction 3575)
        (junction 3580) -> (junction 3596)
        (junction 3578) -> (junction 3580)
        (junction 3575) -> (junction 3581)
    state Init
      entry:
      ChItCtr = 0;
      SlaveNoResponse = 0;
      st_ACChrgModeSt = 0;
      st_DCChrgModeSt = 0;
      st_AcHeatModeSt = 0;
      st_DCHeatModeSt = 0;
      st_DrvOnModeSt = 0;
      bool_DcDcEn = false;
      bool_AcPwrEnbl = false;
      bool_PtcPwrEnbl = false;
      st_ChrgrCmd = ChrgrCmdTyp.IDLE;
      st_EgyCoorrSts = PUDCoorrStsTyp.PUD_Init;
      settings: description=HV off state. BMS is in HVoff or Shutdown state, depending on the operation mode (clamp status). If ignition is off the BMS is commanded to shutdown, if ignition is on it only goes to HVoff. This decision is made in the SetBMSCmd function.
    state ACHeat
      state ACHeat_Init
        entry:
        st_ChrgrCmd = ChrgrCmdTyp.STOP;
        bool_DcDcEn = false;
        bool_AcPwrEnbl = false;
        bool_PtcPwrEnbl = false;
        st_AcHeatModeSt = ACHeatModeTyp.PUD_ACHeat_Init;
        ChItCtr = 0;
        SlaveNoResponse = 0;
      state ACHeat_On
        settings: description=Charging control superstate.
        state ChargingInterrupted
          entry:
          ChItCtr = ChItCtr + 1;
          bool_DcDcEn = false;
          bool_PtcPwrEnbl = false;
          bool_AcPwrEnbl = false;
          st_ChrgrCmd = ChrgrCmdTyp.STOP;
        state ChargerInit
        state ACHeatPhase1
          entry:
          st_ChrgrCmd = ChrgrCmdTyp.ACHeat_PHASE1;
        state HVOFF
          entry:
          st_BmsReq = uint8(BMSCmdTyp.BMS_CMD_HVOFF);
        state ACHeatPhase2
          entry:
          st_ChrgrCmd = uint8(ChrgrCmdTyp.ACHeat_PHASE2);
        state BmsACHeatOn
          entry:
          st_BmsReq = uint8(BMSCmdTyp.BMS_CMD_ACHeatOn);
        state PtcEna
          entry:
          bool_PtcPwrEnbl = true;
        state DcDcEna
          entry:
          bool_DcDcEn = true;
        state ACHeating
          settings: description=Charging control superstate.
          state Heating
            entry:
            st_AcHeatModeSt = ACHeatModeTyp.PUD_ACHeat_On;
            st_EgyCoorrSts = PUDCoorrStsTyp.PUD_ACHeatOn;
            settings: description=Normal charging operation. Charger mains maximum current and target voltage are set and charger is commanded to Active state on entry. Charger output current is computed dynamically according current BMS charging limitations. Start of charging is indicated acoustically by the buzzer.
          ACHeating -> ACHeating [order 1] : after(pPUD_s_EgyCoorrDlyRstCtr_C,sec)/ChItCtr = 0;
          (default) -> Normal.ACHeat.ACHeat_On.ACHeating.Heating
        (default) -> Normal.ACHeat.ACHeat_On.ChargerInit
        Normal.ACHeat.ACHeat_On.ChargingInterrupted -> Normal.ACHeat.ACHeat_On.ChargerInit : after(pPUD_s_EgyCoorrChItRecoverDly_C,sec)
        Normal.ACHeat.ACHeat_On.ChargerInit -> ACHeatPhase1
        ACHeatPhase1 -> Normal.ACHeat.ACHeat_On.ChargingInterrupted [order 1] : after(pPUD_s_ACChrg1NoRespTiout_C,sec)
        ACHeatPhase1 -> Normal.ACHeat.ACHeat_On.HVOFF [order 2] : [st_ChrgrSts == ChrgrStsTyp.CST_ACHeat_PHASE1]
        Normal.ACHeat.ACHeat_On.HVOFF -> Normal.ACHeat.ACHeat_On.ChargingInterrupted [order 1] : after(pPUD_s_EgyCoorrNoRespTiout_C,sec)
        Normal.ACHeat.ACHeat_On.HVOFF -> ACHeatPhase2 [order 2] : [st_BmsSts == BMSStsTyp.BMS_HVOFF_OK]
        ACHeatPhase2 -> Normal.ACHeat.ACHeat_On.ChargingInterrupted [order 1] : after(pPUD_s_ACChrg2NoRespTiout_C,sec)
        ACHeatPhase2 -> BmsACHeatOn [order 2] : [st_ChrgrSts == ChrgrStsTyp.CST_ACHeat_PHASE2]
        BmsACHeatOn -> Normal.ACHeat.ACHeat_On.ChargingInterrupted [order 2] : after(pPUD_s_EgyCoorrNoRespTiout_C,sec)
        BmsACHeatOn -> PtcEna [order 1] : [st_BmsSts == BMSStsTyp.BMS_ACHeatOn]
        PtcEna -> Normal.ACHeat.ACHeat_On.ChargingInterrupted [order 2] : [after(pPUD_s_ACChrgPtcEnDly_C,sec) && ...
            |  V_MCU1MotCapVolt < pPUD_V_MotPwrVolt_C]
        PtcEna -> DcDcEna [order 1] : [after(pPUD_s_ACChrgPtcEnDly_C,sec) && ...
            |  V_MCU1MotCapVolt > pPUD_V_MotPwrVolt_C]
        DcDcEna -> Normal.ACHeat.ACHeat_On.ChargingInterrupted [order 1] : after(pPUD_s_EgyCoorrNoRespTiout_C,sec)
        DcDcEna -> ACHeating [order 2] : [st_DcDcActSts == DCDCAStsTyp.DST_Working]
        ACHeating -> Normal.ACHeat.ACHeat_On.ChargingInterrupted [order 1] : [st_ChrgrSts == ChrgrStsTyp.CST_STOP]
      state ACHeat_Error
        entry:
        st_AcHeatModeSt = ACHeatModeTyp.PUD_ACHeat_Err;
        settings: description=Irrecoverable error state. This state is entered from any other state in the case of irrecoverable error and can only be left back into the HVoff state by resetting Clamp15 (ignition).
      (default) -> ACHeat_Init
      ACHeat_Init -> ACHeat_On
      ACHeat_On -> ACHeat_Error : [ChItCtr > pPUD_cnt_ACHeatItErrThd_C]
    state ACChrg
      state Init
        entry:
        st_ChrgrCmd = ChrgrCmdTyp.STOP;
        bool_DcDcEn = false;
        bool_AcPwrEnbl = false;
        bool_PtcPwrEnbl = false;
        ChItCtr = 0;
        SlaveNoResponse = 0;
        st_ACChrgModeSt = ACChrgModeTyp.PUD_ACChrg_Init;
      state ACChrg
        settings: description=Charging control superstate.
        state ACChargingInterrupted
          entry:
          ChItCtr = ChItCtr + 1;
          bool_DcDcEn = false;
          bool_AcPwrEnbl = false;
          bool_PtcPwrEnbl = false;
          st_ChrgrCmd = uint8(ChrgrCmdTyp.STOP);
        state ChrgInit
        state ChrgCheck
          entry:
          st_ChrgrCmd = uint8(ChrgrCmdTyp.ACChrg_PHASE1);
        state BmsACChrgOn
          entry:
          st_BmsReq = uint8(BMSCmdTyp.BMS_CMD_ACChrgOn);
        state BmsOkDcDcOnAcOn
          entry:
          bool_DcDcEn = true;
          bool_AcPwrEnbl = true;
        state ACChrgPhase2
          entry:
          st_ChrgrCmd = uint8(ChrgrCmdTyp.ACChrg_PHASE2);
        state ACCharging
          settings: description=Charging control superstate.
          state Charging
            entry:
            st_ACChrgModeSt = ACChrgModeTyp.PUD_ACChrg_On;
            st_EgyCoorrSts = PUDCoorrStsTyp.PUD_ACChrgOn;
            settings: description=Normal charging operation. Charger mains maximum current and target voltage are set and charger is commanded to Active state on entry. Charger output current is computed dynamically according current BMS charging limitations. Start of charging is indicated acoustically by the buzzer.
          ACCharging -> ACCharging [order 1] : after(pPUD_s_EgyCoorrDlyRstCtr_C,sec)/ChItCtr = 0;
          (default) -> Normal.ACChrg.ACChrg.ACCharging.Charging
        (default) -> ChrgInit
        ACChargingInterrupted -> ChrgInit : after(pPUD_s_EgyCoorrChItRecoverDly_C,sec)
        ChrgInit -> ChrgCheck
        ChrgCheck -> ACChargingInterrupted [order 2] : after(pPUD_s_ACChrg1NoRespTiout_C,sec)
        ChrgCheck -> BmsACChrgOn [order 1] : [st_ChrgrSts == ChrgrStsTyp.CST_ACChrg_PHASE1]
        BmsACChrgOn -> ACChargingInterrupted [order 2] : after(pPUD_s_EgyCoorrNoRespTiout_C,sec)
        BmsACChrgOn -> Normal.ACChrg.ACChrg.BmsOkDcDcOnAcOn [order 1] : [st_BmsSts == BMSStsTyp.BMS_ACChrgOn]
        Normal.ACChrg.ACChrg.BmsOkDcDcOnAcOn -> ACChargingInterrupted [order 2] : after(pPUD_s_EgyCoorrNoRespTiout_C,sec)
        Normal.ACChrg.ACChrg.BmsOkDcDcOnAcOn -> ACChrgPhase2 [order 1] : [st_DcDcActSts == DCDCAStsTyp.DST_Working]
        ACChrgPhase2 -> ACChargingInterrupted [order 2] : after(pPUD_s_ACChrg2NoRespTiout_C,sec)
        ACChrgPhase2 -> ACCharging [order 1] : [st_ChrgrSts == ChrgrStsTyp.CST_ACChrg_PHASE2]
        ACCharging -> ACChargingInterrupted [order 1] : [st_ChrgrSts == ChrgrStsTyp.CST_STOP]
      state ACChrgError
        entry:
        st_ACChrgModeSt = ACChrgModeTyp.PUD_ACChrg_Err;
        settings: description=Irrecoverable error state. This state is entered from any other state in the case of irrecoverable error and can only be left back into the HVoff state by resetting Clamp15 (ignition).
      (default) -> Normal.ACChrg.Init
      Normal.ACChrg.Init -> Normal.ACChrg.ACChrg
      Normal.ACChrg.ACChrg -> ACChrgError : [ChItCtr > pPUD_cnt_ACChItErrThd_C]
    state DCHeat
      settings: description=Charging control superstate.
      state DCHeat_Init
        entry:
        st_ChrgrCmd = ChrgrCmdTyp.STOP;
        st_DCChrgModeSt = DCHeatModeTyp.PUD_DCHeat_Init;
        bool_DcDcEn = false;
        bool_AcPwrEnbl = false;
        bool_PtcPwrEnbl = false;
        ChItCtr = 0;
        SlaveNoResponse = 0;
      state DCHeat_On
        settings: description=Charging control superstate.
        state DCHeatingInterrupted
          entry:
          ChItCtr = ChItCtr + 1;
          bool_DcDcEn = false;
          bool_AcPwrEnbl = false;
          bool_PtcPwrEnbl = false;
          st_ChrgrCmd = uint8(ChrgrCmdTyp.STOP);
        state ChargerInit
        state DCHeatPhase1
          entry:
          st_ChrgrCmd = uint8(ChrgrCmdTyp.DCHeat_PHASE1);
        state HVOFF
          entry:
          st_BmsReq = uint8(BMSCmdTyp.BMS_CMD_HVOFF);
        state DCHeatPhase2
          entry:
          st_ChrgrCmd = uint8(ChrgrCmdTyp.DCHeat_PHASE2);
        state BmsDCHeatOn
          entry:
          st_BmsReq = uint8(BMSCmdTyp.BMS_CMD_DCHeatOn);
        state BmsOkDcDcOn
          entry:
          bool_DcDcEn = true;
        state DcDcOKPtcOn
          entry:
          bool_PtcPwrEnbl = true;
        state DCHeating
          settings: description=Charging control superstate.
          state Heating
            entry:
            st_DCHeatModeSt = DCHeatModeTyp.PUD_DCHeat_On;
            st_EgyCoorrSts = PUDCoorrStsTyp.PUD_DCHeatOn;
            settings: description=Normal charging operation. Charger mains maximum current and target voltage are set and charger is commanded to Active state on entry. Charger output current is computed dynamically according current BMS charging limitations. Start of charging is indicated acoustically by the buzzer.
          DCHeating -> DCHeating [order 1] : after(pPUD_s_EgyCoorrDlyRstCtr_C,sec)/ChItCtr = 0;
          (default) -> Normal.DCHeat.DCHeat_On.DCHeating.Heating
        (default) -> Normal.DCHeat.DCHeat_On.ChargerInit
        DCHeatingInterrupted -> Normal.DCHeat.DCHeat_On.ChargerInit : after(pPUD_s_EgyCoorrChItRecoverDly_C,sec)
        Normal.DCHeat.DCHeat_On.ChargerInit -> DCHeatPhase1
        DCHeatPhase1 -> DCHeatingInterrupted [order 1] : after(pPUD_s_DCChrg1NoRespTiout_C,sec)
        DCHeatPhase1 -> Normal.DCHeat.DCHeat_On.HVOFF [order 2] : [st_ChrgrSts == ChrgrStsTyp.CST_DCHeat_PHASE1]
        Normal.DCHeat.DCHeat_On.HVOFF -> DCHeatingInterrupted [order 2] : after(pPUD_s_EgyCoorrNoRespTiout_C,sec)
        Normal.DCHeat.DCHeat_On.HVOFF -> DCHeatPhase2 [order 1] : [st_BmsSts == BMSStsTyp.BMS_HVOFF_OK]
        DCHeatPhase2 -> DCHeatingInterrupted [order 1] : after(pPUD_s_DCChrg2NoRespTiout_C,sec)
        DCHeatPhase2 -> BmsDCHeatOn [order 2] : [st_ChrgrSts == ChrgrStsTyp.CST_DCHeat_PHASE2]
        BmsDCHeatOn -> DCHeatingInterrupted [order 1] : after(pPUD_s_BMSOnNoRespTiout_C,sec)
        BmsDCHeatOn -> BmsOkDcDcOn [order 2] : [st_BmsSts == BMSStsTyp.BMS_DCHeatOn]
        BmsOkDcDcOn -> DCHeatingInterrupted [order 1] : after(pPUD_s_EgyCoorrNoRespTiout_C,sec)
        BmsOkDcDcOn -> DcDcOKPtcOn [order 2] : [st_DcDcActSts == DCDCAStsTyp.DST_Working]
        DcDcOKPtcOn -> DCHeating
        DCHeating -> DCHeatingInterrupted [order 1] : [st_ChrgrSts == ChrgrStsTyp.CST_STOP]
      state DCHeat_Err
        entry:
        st_DCHeatModeSt = DCHeatModeTyp.PUD_DCHeat_Err;
        settings: description=Irrecoverable error state. This state is entered from any other state in the case of irrecoverable error and can only be left back into the HVoff state by resetting Clamp15 (ignition).
      (default) -> DCHeat_Init
      DCHeat_Init -> DCHeat_On
      DCHeat_On -> DCHeat_Err : [ChItCtr > pPUD_cnt_DCHeatItErrThd_C]
    state DCChrg
      settings: description=Charging control superstate.
      state DCChrg_Init
        entry:
        st_ChrgrCmd = ChrgrCmdTyp.STOP;
        st_DCChrgModeSt = DCChrgModeTyp.PUD_DCChrg_Init;
        bool_DcDcEn = false;
        bool_AcPwrEnbl = false;
        bool_PtcPwrEnbl = false;
        ChItCtr = 0;
        SlaveNoResponse = 0;
      state DCChrg_On
        settings: description=Charging control superstate.
        state ChargingInterrupted
          entry:
          ChItCtr = ChItCtr + 1;
          bool_DcDcEn = false;
          bool_AcPwrEnbl = false;
          bool_PtcPwrEnbl = false;
          st_ChrgrCmd = uint8(ChrgrCmdTyp.STOP);
        state ChargerInit
        state DCChrgPhase1
          entry:
          st_ChrgrCmd = uint8(ChrgrCmdTyp.DCChrg_PHASE1);
        state BmsDCChrgOn
          entry:
          st_BmsReq = uint8(BMSCmdTyp.BMS_CMD_DCChrgOn);
        state BmsOkDcDcOnAcOn
          entry:
          bool_DcDcEn = true;
          bool_AcPwrEnbl = true;
        state DCChrgPhase2
          entry:
          st_ChrgrCmd = uint8(ChrgrCmdTyp.DCChrg_PHASE2);
        state DCChrging
          settings: description=Charging control superstate.
          state Charging
            entry:
            st_DCChrgModeSt = DCChrgModeTyp.PUD_DCChrg_On;
            st_EgyCoorrSts = PUDCoorrStsTyp.PUD_DCChrgOn;
            settings: description=Normal charging operation. Charger mains maximum current and target voltage are set and charger is commanded to Active state on entry. Charger output current is computed dynamically according current BMS charging limitations. Start of charging is indicated acoustically by the buzzer.
          DCChrging -> DCChrging [order 1] : after(pPUD_s_EgyCoorrDlyRstCtr_C,sec)/ChItCtr = 0;
          (default) -> Normal.DCChrg.DCChrg_On.DCChrging.Charging
        (default) -> Normal.DCChrg.DCChrg_On.ChargerInit
        Normal.DCChrg.DCChrg_On.ChargingInterrupted -> Normal.DCChrg.DCChrg_On.ChargerInit : after(pPUD_s_EgyCoorrChItRecoverDly_C,sec)
        Normal.DCChrg.DCChrg_On.ChargerInit -> DCChrgPhase1
        DCChrgPhase1 -> Normal.DCChrg.DCChrg_On.ChargingInterrupted [order 1] : after(pPUD_s_DCChrg1NoRespTiout_C,sec)
        DCChrgPhase1 -> BmsDCChrgOn [order 2] : [st_ChrgrSts == ChrgrStsTyp.CST_DCChrg_PHASE1]
        BmsDCChrgOn -> Normal.DCChrg.DCChrg_On.ChargingInterrupted [order 2] : after(pPUD_s_EgyCoorrNoRespTiout_C,sec)
        BmsDCChrgOn -> Normal.DCChrg.DCChrg_On.BmsOkDcDcOnAcOn [order 1] : [st_BmsSts == BMSStsTyp.BMS_DCChrgOn]
        Normal.DCChrg.DCChrg_On.BmsOkDcDcOnAcOn -> Normal.DCChrg.DCChrg_On.ChargingInterrupted [order 2] : after(pPUD_s_EgyCoorrNoRespTiout_C,sec)
        Normal.DCChrg.DCChrg_On.BmsOkDcDcOnAcOn -> DCChrgPhase2 [order 1] : [st_DcDcActSts == DCDCAStsTyp.DST_Working]
        DCChrgPhase2 -> Normal.DCChrg.DCChrg_On.ChargingInterrupted [order 2] : after(pPUD_s_DCChrg2NoRespTiout_C,sec)
        DCChrgPhase2 -> DCChrging [order 1] : [st_ChrgrSts == ChrgrStsTyp.CST_DCChrg_PHASE2]
        DCChrging -> Normal.DCChrg.DCChrg_On.ChargingInterrupted [order 1] : [st_ChrgrSts == ChrgrStsTyp.CST_STOP]
      state DCChrg_Err
        entry:
        st_DCChrgModeSt = DCChrgModeTyp.PUD_DCChrg_Err;
        settings: description=Irrecoverable error state. This state is entered from any other state in the case of irrecoverable error and can only be left back into the HVoff state by resetting Clamp15 (ignition).
      (default) -> DCChrg_Init
      DCChrg_Init -> DCChrg_On
      DCChrg_On -> DCChrg_Err : [ChItCtr > pPUD_cnt_DCChItErrThd_C]
    state Drv
      exit:
      st_DrvOnModeSt = DrvOnModeTyp.PUD_DrvOn_Init;
      settings: description=BMS HVon state.
      state DrvOn
        state DrvOn_Init
          entry:
          st_ChrgrCmd = ChrgrCmdTyp.STOP;
          bool_DcDcEn = false;
          bool_AcPwrEnbl = false;
          bool_PtcPwrEnbl = false;
          ChItCtr = 0;
          SlaveNoResponse = 0;
          st_DrvOnModeSt = DrvOnModeTyp.PUD_DrvOn_Init;
        state DrvOn_On
          en:
          st_EgyCoorrSts = PUDCoorrStsTyp.PUD_DrvOn;
          state ChargerInit
          state HvOn_Failed
            entry:
            ChItCtr = ChItCtr + 1;
            st_ChrgrCmd = uint8(ChrgrCmdTyp.STOP);
          state BMSOn
            entry:
            st_BmsReq = uint8(BMSCmdTyp.BMS_CMD_HVOn);
          state BmsOk_DcDcOnAcOn
            entry:
            bool_DcDcEn = true;
            bool_AcPwrEnbl = true;
            bool_PtcPwrEnbl = true;
          state HvOn
            entry:
            st_DrvOnModeSt = DrvOnModeTyp.PUD_DrvOn_Ok;
            st_EgyCoorrSts = PUDCoorrStsTyp.PUD_DrvOn;
          (default) -> Normal.Drv.DrvOn.DrvOn_On.ChargerInit
          Normal.Drv.DrvOn.DrvOn_On.ChargerInit -> BMSOn
          BMSOn -> HvOn_Failed [order 2] : after(pPUD_s_EgyCoorrNoRespTiout_C,sec)
          BMSOn -> BmsOk_DcDcOnAcOn [order 1] : [st_BmsSts == BMSStsTyp.BMS_HVOn]
          BmsOk_DcDcOnAcOn -> HvOn
        state DrvOn_Err
          entry:
          st_DrvOnModeSt = DrvOnModeTyp.PUD_DrvOn_Err;
          settings: description=Irrecoverable error state. This state is entered from any other state in the case of irrecoverable error and can only be left back into the HVoff state by resetting Clamp15 (ignition).
        (default) -> DrvOn_Init
        DrvOn_Init -> DrvOn_On
        DrvOn_On -> DrvOn_Err : [ChItCtr > 0]
      state DrvErr
        state Init
          entry:
          bool_DcDcEn = false;
          bool_AcPwrEnbl = false;
          bool_PtcPwrEnbl = false;
          ChItCtr = 0;
          SlaveNoResponse = 0;
        state Motor_ShtDwn
        state DcDcOffOk_BmsOffAcOff
          entry:
          st_BmsReq = uint8(BMSCmdTyp.BMS_CMD_HVOFF);
        state HvOff
          entry:
          st_EgyCoorrSts = PUDCoorrStsTyp.PUD_DrvErr;
        (default) -> Normal.Drv.DrvErr.Init
        Normal.Drv.DrvErr.Init -> Normal.Drv.DrvErr.Motor_ShtDwn : [st_DcDcActSts ==DCDCAStsTyp.DST_ShutDown && ...
            | bool_HvPwrOffEnbl == true || ...
            | after(pPUD_s_EgyCoorrNoRespTiout_C,sec)]
        Normal.Drv.DrvErr.Motor_ShtDwn -> DcDcOffOk_BmsOffAcOff : [bool_MotShtdwnAllow == true]
        DcDcOffOk_BmsOffAcOff -> Normal.Drv.DrvErr.HvOff : [st_BmsSts == BMSStsTyp.BMS_HVOFF_OK]
      DrvErr -> DrvOn : [st_PUDCoorrReq == PUDCoorrStsTyp.PUD_DrvOn]
      (default) -> DrvOn
      DrvOn -> DrvErr : [st_PUDCoorrReq == PUDCoorrStsTyp.PUD_DrvErr]
    (default) -> Normal.Init
    ACHeat -> HVOff [order 1] : [st_PUDCoorrReq == PUDCoorrStsTyp.PUD_HVOFF]
    Normal.Init -> ACHeat [order 6] : [st_PUDCoorrReq == PUDCoorrStsTyp.PUD_ACHeatOn]
    HVOff -> ACHeat [order 5] : [st_PUDCoorrReq == PUDCoorrStsTyp.PUD_ACHeatOn]
    Normal.ACChrg -> ACHeat [order 2] : [st_PUDCoorrReq == PUDCoorrStsTyp.PUD_ACHeatOn]
    ACHeat -> Normal.ACChrg [order 2] : [st_PUDCoorrReq == PUDCoorrStsTyp.PUD_ACChrgOn]
    Normal.Init -> Normal.ACChrg [order 3] : [st_PUDCoorrReq == PUDCoorrStsTyp.PUD_ACChrgOn]
    Normal.ACChrg -> HVOff [order 1] : [st_PUDCoorrReq == PUDCoorrStsTyp.PUD_HVOFF]
    HVOff -> Normal.ACChrg [order 1] : [st_PUDCoorrReq == PUDCoorrStsTyp.PUD_ACChrgOn]
    DCHeat -> HVOff [order 1] : [st_PUDCoorrReq == PUDCoorrStsTyp.PUD_HVOFF]
    HVOff -> DCHeat [order 4] : [st_PUDCoorrReq == PUDCoorrStsTyp.PUD_DCHeatOn]
    Normal.Init -> DCHeat [order 5] : [st_PUDCoorrReq == PUDCoorrStsTyp.PUD_DCHeatOn]
    DCChrg -> DCHeat [order 2] : [st_PUDCoorrReq == PUDCoorrStsTyp.PUD_DCHeatOn]
    DCHeat -> DCChrg [order 2] : [st_PUDCoorrReq == PUDCoorrStsTyp.PUD_DCChrgOn]
    DCChrg -> HVOff [order 1] : [st_PUDCoorrReq == PUDCoorrStsTyp.PUD_HVOFF]
    Normal.Init -> DCChrg [order 2] : [st_PUDCoorrReq == PUDCoorrStsTyp.PUD_DCChrgOn]
    HVOff -> DCChrg [order 3] : [st_PUDCoorrReq == PUDCoorrStsTyp.PUD_DCChrgOn]
    Drv -> HVOff : [st_PUDCoorrReq == PUDCoorrStsTyp.PUD_HVOFF]
      settings: description=Go to the HVoff state if BMS is in HVoff, Shutdown or Charging state. In case of charging, the machine will transit to the charging state through the HVOff state.
    Normal.Init -> Drv [order 1] : [st_PUDCoorrReq == PUDCoorrStsTyp.PUD_DrvOn]
      settings: description=Transit to HVon state of the BMS status changes to HVon.
    HVOff -> Drv [order 2] : [st_PUDCoorrReq == PUDCoorrStsTyp.PUD_DrvOn]
    Normal.Init -> HVOff [order 4] : [st_PUDCoorrReq == PUDCoorrStsTyp.PUD_HVOFF]
  state EmgHVOff
    en:
    st_EgyCoorrSts = PUDCoorrStsTyp.PUD_EmgHVOFF;
    settings: description=Irrecoverable error state. This state is entered from any other state in the case of irrecoverable error and can only be left back into the HVoff state by resetting Clamp15 (ignition).
    state Motor_STOP
      entry:
      bool_DcDcEn = false;
      bool_AcPwrEnbl = false;
      bool_PtcPwrEnbl = false;
      st_ChrgrCmd = ChrgrCmdTyp.STOP;
    state BMS_HVOFF
      en:
      st_BmsReq = BMSCmdTyp.BMS_CMD_EmgHVOFF;
    state HvOff_ERR
      entry:
      st_EgyCoorrSts = PUDCoorrStsTyp.PUD_EmgHVOFF_ERR;
    state RapidDischarge
      entry:
      bool_RpdDisChrgPerm = true;
    state HVOFF_OK
      en:
      st_EgyCoorrSts = PUDCoorrStsTyp.PUD_EmgHVOFF_OK;
    (default) -> Motor_STOP
    Motor_STOP -> BMS_HVOFF
    BMS_HVOFF -> EmgHVOff.HvOff_ERR [order 2] : [st_BmsSts == BMSStsTyp.BMS_EmgHVOFF_ERR]
    BMS_HVOFF -> EmgHVOff.RapidDischarge [order 1] : [st_BmsSts == BMSStsTyp.BMS_EmgHVOFF_OK]
    EmgHVOff.HvOff_ERR -> HVOFF_OK : [V_MCU1MotCapVolt < pPUD_V_MotRpdDisVolt_C && ...
        | V_MCU2MotCapVolt < pPUD_V_MotRpdDisVolt_C ]
    EmgHVOff.RapidDischarge -> HVOFF_OK : [V_MCU1MotCapVolt < pPUD_V_MotRpdDisVolt_C && ...
        | V_MCU2MotCapVolt < pPUD_V_MotRpdDisVolt_C ]
  (default) -> Normal
  Normal -> EmgHVOff : [st_PUDCoorrReq == PUDCoorrStsTyp.PUD_EmgHVOFF]
  data: st_PUDCoorrReq input; bool_MotShtdwnAllow input; V_MCU1MotCapVolt input; V_MCU2MotCapVolt input; bool_HvPwrOffEnbl input; bool_ACChrgrPlugDtctd input; bool_DCChrgrPlugDtctd input; st_BmsSts input; st_ChrgrSts input; st_DcDcActSts input; st_EgyCoorrSts output uint8 =PUDCoorrStsTyp.PUD_HVOFF; st_BmsReq output uint8 =BMSCmdTyp.BMS_CMD_IDLE; st_ChrgrCmd output uint8; bool_DcDcEn output boolean =0; SlaveNoResponse local boolean =0; pPUD_s_EgyCoorrNoRespTiout_C input =0.5; ChItCtr local uint8; pPUD_s_EgyCoorrChItRecoverDly_C input; pPUD_s_EgyCoorrDlyRstCtr_C input; bool_AcPwrEnbl output boolean; st_ACChrgModeSt output uint8; st_DCChrgModeSt output uint8; st_AcHeatModeSt output uint8; st_DCHeatModeSt output uint8; st_DrvOnModeSt output uint8; bool_PtcPwrEnbl output boolean; bool_RpdDisChrgPerm output boolean; pPUD_V_MotRpdDisVolt_C input; pPUD_s_DCChrg1NoRespTiout_C input; pPUD_s_BMSOnNoRespTiout_C input; pPUD_s_ACChrg1NoRespTiout_C input; pPUD_s_ACChrg2NoRespTiout_C input; pPUD_s_DCChrg2NoRespTiout_C input; pPUD_cnt_ACChItErrThd_C input; pPUD_cnt_DCChItErrThd_C input; pPUD_cnt_ACHeatItErrThd_C input; pPUD_cnt_DCHeatItErrThd_C input; pPUD_V_MotPwrVolt_C input; pPUD_s_ACChrgPtcEnDly_C input
